simulink model "ofb"  (Simulink 7.8)
settings: Solver=ode45  StartTime=0.0  StopTime=1e-1  RelTol=1e-3
values from neighbouring files (symbols this model uses):
  corrmagnetgain = param.corrmagnetgain    [simofb.m]
  s2ffactor = param.s2ffactor    [simofb.m]
  Ts = param.Ts    [simofb.m]    (also in simofbuvx.m = 0.00032)
undefined symbols (not defined in the file or in its folder): fracdelay
libraries: cstblocks x8
settings Model: Creator=daniel.tavares  LastModifiedBy=danielot
settings DataIOCC: ExternalInput=[simvectors.t simvectors.reference_orbit simvectors.orbit_distortion simvectors.fofb_setpoints simvectors.bpm_noise simvectors.sofb_setpoints simvectors.corrsofb_current_noise simvectors.corrsofb_power_noise]  LimitDataPoints=off  LoadExternalInput=on  SaveFormat=StructureWithTime  SignalLogging=off  DSMLogging=off
settings DebuggingCC: AlgebraicLoopMsg=none  ArtificialAlgebraicLoopMsg=none  ModelReferenceExtraNoncontSigs=none

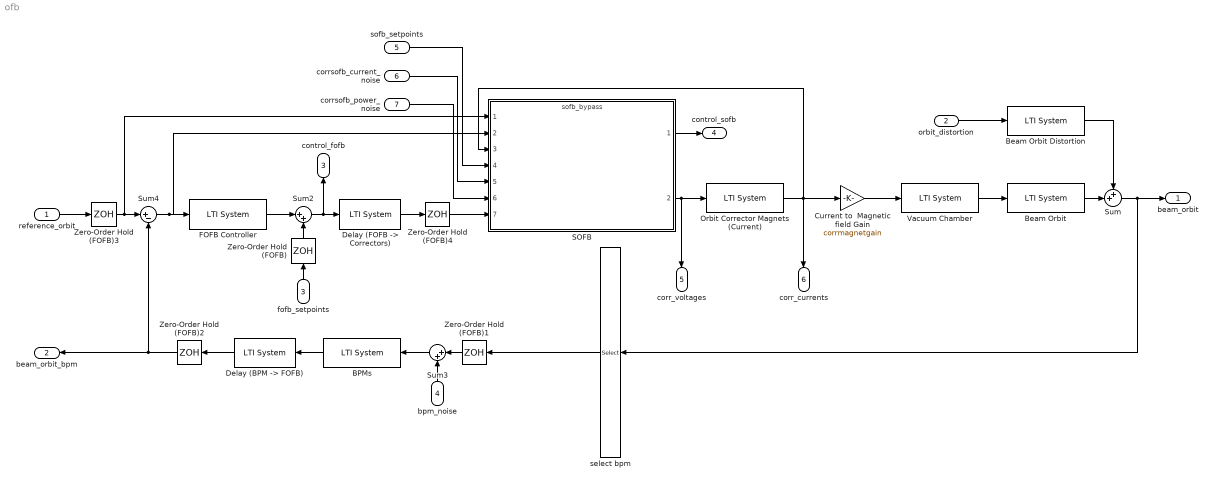
== system ofb ==
  reference_orbit : Inport  PortDimensions=nbpm  SampleTime=Ts
  orbit_distortion : Inport  Port=2  PortDimensions=ndist
  fofb_setpoints : Inport  Port=3  PortDimensions=ncorrfofb
  bpm_noise : Inport  Port=4  PortDimensions=nbpm
  sofb_setpoints : Inport  Port=5  PortDimensions=ncorrsofb  SampleTime=Ts*s2ffactor
  corrsofb_current_noise : Inport  Port=6  PortDimensions=ncorrsofb  SampleTime=0
  corrsofb_power_noise : Inport  Port=7  PortDimensions=ncorrsofb  SampleTime=0
  BPMs : cstblocks/LTI System  sys=bpm  IC=[]
  Beam Orbit : cstblocks/LTI System  sys=beam  IC=[]
  Beam Orbit Distortion : cstblocks/LTI System  sys=distbeam  IC=[]
  Current to  Magnetic field Gain : Gain  Gain=corrmagnetgain
  "Delay (BPM -> FOFB)" : cstblocks/LTI System  sys=delay.bpm  IC=[]
  "Delay (FOFB -> Correctors)" : cstblocks/LTI System  sys=delay.corrfofb  IC=[]
  FOFB Controller : cstblocks/LTI System  sys=fofbctrl  IC=[]
  Orbit Corrector Magnets (Current) : cstblocks/LTI System  sys=corrmagnet  IC=[]
  SOFB : ModelReference  ModelNameDialog=sofb_bypass.mdl  SimulationMode=Normal  ModelReferenceVersion=1.31  CopyOfModelName=sofb_bypass.mdl  DefaultDataLogging=on
  Sum : Sum  Inputs=++|
  Sum2 : Sum  Inputs=|++
  Sum3 : Sum  Inputs=|++
  Sum4 : Sum  Inputs=|+-
  Vacuum Chamber : cstblocks/LTI System  sys=vacchamb  IC=[]
  Zero-Order Hold (FOFB) : ZeroOrderHold  SampleTime=[Ts fracdelay.bpm]
  Zero-Order Hold (FOFB)1 : ZeroOrderHold  SampleTime=Ts
  Zero-Order Hold (FOFB)2 : ZeroOrderHold  SampleTime=[Ts fracdelay.bpm]
  Zero-Order Hold (FOFB)3 : ZeroOrderHold  SampleTime=[Ts fracdelay.bpm]
  Zero-Order Hold (FOFB)4 : ZeroOrderHold  SampleTime=[Ts (fracdelay.bpm+fracdelay.corrfofb)]
  select bpm : Selector  InputPortWidth=norbit  IndexOptions=Index vector (dialog)  Indices=bpmordering  OutputSizes=1
  beam_orbit : Outport
  beam_orbit_bpm : Outport  Port=2
  control_fofb : Outport  Port=3
  control_sofb : Outport  Port=4
  corr_voltages : Outport  Port=5
  corr_currents : Outport  Port=6
  wires:
  Beam Orbit/1 -> Sum/2
  orbit_distortion/1 -> Beam Orbit Distortion/1
  bpm_noise/1 -> Sum3/2
  Vacuum Chamber/1 -> Beam Orbit/1
  Beam Orbit Distortion/1 -> Sum/1
  Sum/1 -> beam_orbit/1, select bpm/1
  Orbit Corrector Magnets (Current)/1 -> Current to  Magnetic field Gain/1, corr_currents/1, SOFB/3
  reference_orbit/1 -> Zero-Order Hold (FOFB)3/1
  fofb_setpoints/1 -> Zero-Order Hold (FOFB)/1
  Zero-Order Hold (FOFB)/1 -> Sum2/2
  Zero-Order Hold (FOFB)2/1 -> beam_orbit_bpm/1, Sum4/2
  Sum4/1 -> SOFB/2, FOFB Controller/1
  Zero-Order Hold (FOFB)4/1 -> SOFB/7
  "Delay (FOFB -> Correctors)"/1 -> Zero-Order Hold (FOFB)4/1
  BPMs/1 -> "Delay (BPM -> FOFB)"/1
  "Delay (BPM -> FOFB)"/1 -> Zero-Order Hold (FOFB)2/1
  FOFB Controller/1 -> Sum2/1
  Sum2/1 -> "Delay (FOFB -> Correctors)"/1, control_fofb/1
  SOFB/1 -> control_sofb/1
  sofb_setpoints/1 -> SOFB/4
  corrsofb_current_noise/1 -> SOFB/5
  corrsofb_power_noise/1 -> SOFB/6
  SOFB/2 -> corr_voltages/1, Orbit Corrector Magnets (Current)/1
  Zero-Order Hold (FOFB)3/1 -> Sum4/1, SOFB/1
  Zero-Order Hold (FOFB)1/1 -> Sum3/1
  select bpm/1 -> Zero-Order Hold (FOFB)1/1
  Sum3/1 -> BPMs/1
  Current to  Magnetic field Gain/1 -> Vacuum Chamber/1
